simulink subsystem "s0315_alpha_controller_PP_int"  (R2019b)
settings: Solver=VariableStepAuto  StartTime=0.0  StopTime=10.0  RelTol=1e-3
model mask{p1=0, p2=0, p3=0}
  mask prompts: p1 "Position 1st pole"; p2 "Position 2nd pole"; p3 "Position 3rd pole"
undefined symbols (not defined in the file): DiscIntNeverNeededParam, PARAMS
libraries: simulink x1
settings Model: Creator=francescoceresetti  LastModifiedBy=francescoceresetti

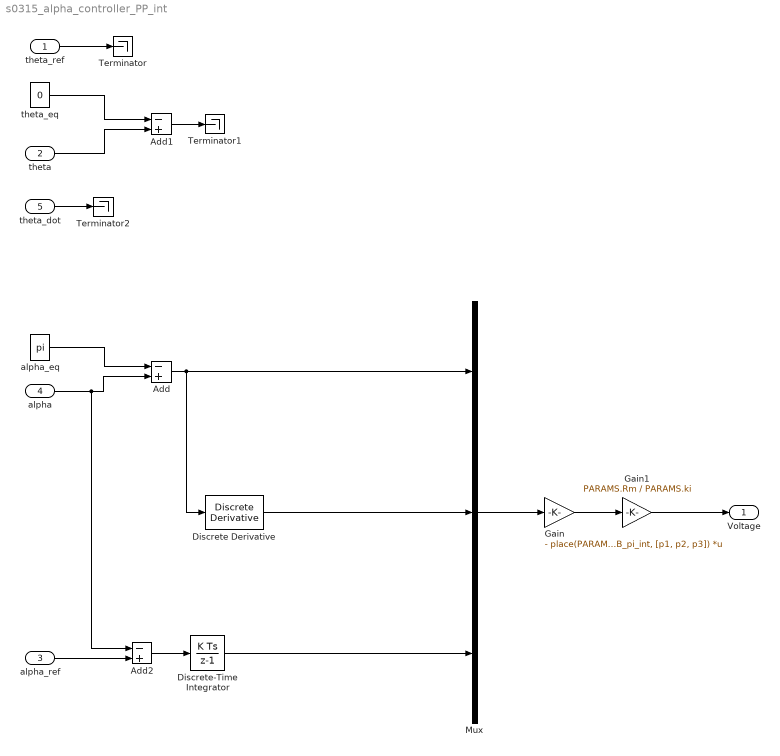
== system s0315_alpha_controller_PP_int ==
  theta_ref : Inport
  theta : Inport  Port=2
  alpha_ref : Inport  Port=3
  alpha : Inport  Port=4
  theta_dot : Inport  Port=5
  Add : Sum  Inputs=-+
  Add1 : Sum  Inputs=-+
  Add2 : Sum  Inputs=-+
  Discrete Derivative : simulink/Discrete/Discrete Derivative  gainval=1.0  ICPrevScaledInput=pi  OutMin=[]  OutMax=[]  OutDataType=fixdt(1, 16)  OutScaling=2^-10  DoSatur=off
  Discrete-Time Integrator : DiscreteIntegrator  SampleTime=-1  ICPrevOutput=DiscIntNeverNeededParam  ICPrevScaledInput=DiscIntNeverNeededParam
  Gain : Gain  Gain=- place(PARAMS.A_pi_int, PARAMS.B_pi_int, [p1, p2, p3])  Multiplication=Matrix(K*u)
  Gain1 : Gain  Gain=PARAMS.Rm / PARAMS.ki
  Mux : Mux  Inputs=3
  Terminator : Terminator
  Terminator1 : Terminator
  Terminator2 : Terminator
  "alpha_eq " : Constant  Value=pi
  theta_eq : Constant  Value=0
  Voltage : Outport
  wires:
  theta_ref/1 -> Terminator/1
  alpha/1 -> Add2/1, Add/2
  Mux/1 -> Gain/1
  Gain/1 -> Gain1/1
  Gain1/1 -> Voltage/1
  "alpha_eq "/1 -> Add/1
  theta_eq/1 -> Add1/1
  theta/1 -> Add1/2
  alpha_ref/1 -> Add2/2
  Add2/1 -> Discrete-Time Integrator/1
  Add1/1 -> Terminator1/1
  theta_dot/1 -> Terminator2/1
  Add/1 -> Mux/1, Discrete Derivative/1
  Discrete-Time Integrator/1 -> Mux/3
  Discrete Derivative/1 -> Mux/2
